simulink model "DLS_Controller_SW"  (Simulink 7.9)
settings: Solver=FixedStepDiscrete  StartTime=0.0  StopTime=10  RelTol=1e-3
PreLoadFcn:
  | DLS_Controller_SW_selfinit
settings Model: Creator=fguerin  LastModifiedBy=klindqvi  RecordCoverage=on
settings DataIOCC: ExternalInput=[t,u]  LimitDataPoints=off  SaveOutput=off  DSMLogging=off  SaveTime=off  SignalLoggingName=logsOut
settings OptimizationCC: InlineParams=on  InlineInvariantSignals=on  EnhancedBackFolding=on  ZeroExternalMemoryAtStartup=off  ZeroInternalMemoryAtStartup=off  EfficientFloat2IntCast=on  OptimizeModelRefInitCode=on  LifeSpan=1
settings DebuggingCC: SignalInfNanChecking=error  SignalRangeChecking=error  ReadBeforeWriteMsg=EnableAllAsError  WriteAfterWriteMsg=EnableAllAsError  WriteAfterReadMsg=EnableAllAsError  AlgebraicLoopMsg=error  ArtificialAlgebraicLoopMsg=error  SaveWithDisabledLinksMsg=error  SaveWithParameterizedLinksMsg=error  CheckExecutionContextPreStartOutputMsg=on  CheckExecutionContextRuntimeOutputMsg=on  BlockPriorityViolationMsg=error  SolverPrmCheckMsg=error  MultiTaskCondExecSysMsg=warning  MultiTaskRateTransMsg=warning  CheckMatrixSingularityMsg=error  IntegerOverflowMsg=error  ParameterUnderflowMsg=error  ParameterPrecisionLossMsg=error  ParameterTunabilityLossMsg=error  UnderSpecifiedDataTypeMsg=warning  UnnecessaryDatatypeConvMsg=warning  VectorMatrixConversionMsg=error  SFcnCompatibilityMsg=error  BusObjectLabelMismatch=error  RootOutportRequireBusObject=error  AssertControl=DisableAll  ModelReferenceIOMsg=error  ModelReferenceIOMismatchMessage=error  ModelReferenceCSMismatchMessage=warning  UnknownTsInhSupMsg=error  ModelReferenceDataLoggingMessage=error  ModelReferenceSymbolNameMessage=none  StrictBusMsg=ErrorOnBusTreatedAsVector
settings HardwareCC: ProdLargestAtomicInteger=Long  ProdLargestAtomicFloat=Double  ProdIntDivRoundTo=Zero  ProdEndianess=BigEndian  ProdHWDeviceType=Freescale->MPC5500
settings ModelReferenceCC: ModelReferenceNumInstancesAllowed=Single
settings SFSimCC: SimParseCustomCode=off
settings RTWCC: SystemTargetFile=ert.tlc  TemplateMakefile=ert_default_tmf  Description=Embedded Coder  GenerateReport=on  RTWVerbose=off  ProcessScript=ert_make_rtw_hook  IncludeHyperlinkInReport=on  LaunchReport=on  GenerateTraceInfo=on  GenerateTraceReport=on  GenerateTraceReportSl=on  GenerateTraceReportSf=on  GenerateTraceReportEml=on  GenerateCodeMetricsReport=on
settings MATStruct: className=rtw.pil.Bullseye  argsAllComponents=[]  excludedModels=[]  includeReferencedModels=off  includeTopModel=on  enabled=off
settings CodeAppCC: ForceParamTrailComments=on  IgnoreCustomStorageClasses=off  IgnoreTestpoints=on  MangleLength=4  InlinedPrmAccess=Macros  ReqsInCode=on
settings ERTTargetCC: CodeReplacementLibrary=ANSI_C  MultiwordLength=2048  GenerateSampleERTMain=on  SupportAbsoluteTime=off  SupportNonFinite=off  SupportComplex=off  PortableWordSizes=on  InlinedParameterPlacement=NonHierarchical  ERTCustomFileTemplate=example_file_process.tlc  ConvertIfToSwitch=off  SuppressUnreachableDefaultCases=off
settings ConfigComp: Description=Design Verifier Custom Configuration Component  DVMaxProcessTime=600  DVDisplayUnsatisfiableObjectives=on  DVAutomaticStubbing=off  DVOutputDir=C:\Work\Data\Pilots\P_PSA_ECoder_BenchMark_LaGarenne\source9b\deliverable\trunk\demos\VnV_example\Projects\ADL_Project/Simulink_Test_Generation/ADL_Sim  DVModelCoverageObjectives=MCDC  DVTestSuiteOptimization=CombinedObjectives  DVDataFileName=./Tests/$ModelName$_sldvdata  DVSaveHarnessModel=on  DVHarnessModelFileName=./Tests/$ModelName$_testHarness  DVModelReferenceHarness=on  DVSaveReport=on  DVReportFileName=ADL_Sim_SLDV.html

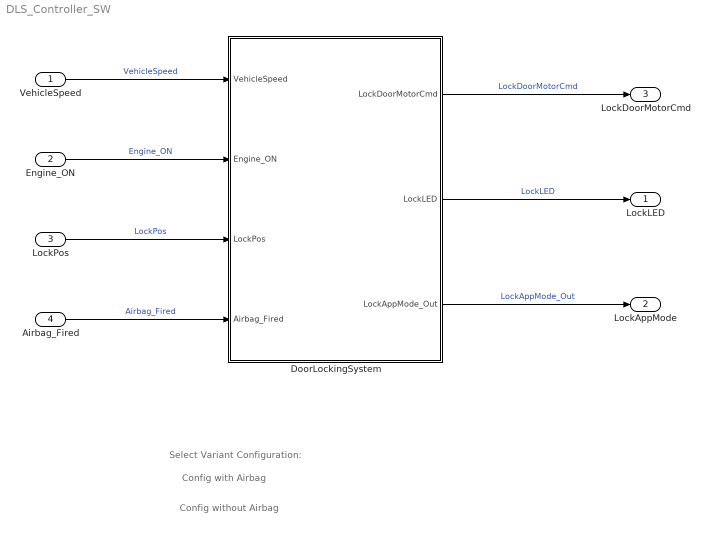
== system DLS_Controller_SW ==
  note: Select Variant Configuration:
  note: Config with Airbag
  note: Config without Airbag
  VehicleSpeed : Inport  PortDimensions=1  SampleTime=0.25
  Engine_ON : Inport  Port=2  PortDimensions=1  SampleTime=0.25
  LockPos : Inport  Port=3  SampleTime=0.25
  Airbag_Fired : Inport  Port=4  OutDataTypeStr=boolean  PortDimensions=1  SampleTime=0.25
  DoorLockingSystem : Subsystem
  LockLED : Outport  OutDataTypeStr=boolean  PortDimensions=1
  LockAppMode : Outport  Port=2
  LockDoorMotorCmd : Outport  Port=3
  wires:
  VehicleSpeed/1 -> DoorLockingSystem/1(VehicleSpeed)  "VehicleSpeed"
  Engine_ON/1 -> DoorLockingSystem/2(Engine_ON)  "Engine_ON"
  DoorLockingSystem/2(LockLED) -> LockLED/1  "LockLED"
  DoorLockingSystem/1(LockDoorMotorCmd) -> LockDoorMotorCmd/1  "LockDoorMotorCmd"
  LockPos/1 -> DoorLockingSystem/3(LockPos)  "LockPos"
  Airbag_Fired/1 -> DoorLockingSystem/4(Airbag_Fired)  "Airbag_Fired"
  DoorLockingSystem/3(LockAppMode_Out) -> LockAppMode/1  "LockAppMode_Out"

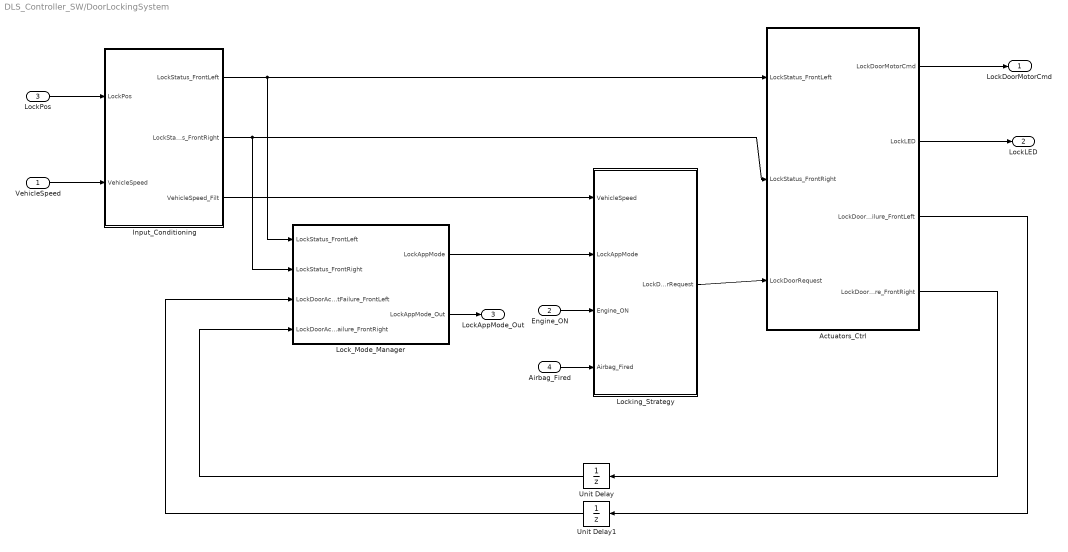
== system DLS_Controller_SW/DoorLockingSystem ==
  VehicleSpeed : Inport
  Engine_ON : Inport  Port=2  PortDimensions=1
  LockPos : Inport  Port=3
  Airbag_Fired : Inport  Port=4  OutDataTypeStr=boolean  PortDimensions=1
  Actuators_Ctrl : Subsystem
  Input_Conditioning : Subsystem
  Lock_Mode_Manager : Subsystem
  Locking_Strategy : Subsystem
  Unit Delay : UnitDelay  SampleTime=-1
  Unit Delay1 : UnitDelay  SampleTime=-1
  LockDoorMotorCmd : Outport
  LockLED : Outport  Port=2
  LockAppMode_Out : Outport  Port=3
  wires:
  VehicleSpeed/1 -> Input_Conditioning/2(VehicleSpeed)
  Engine_ON/1 -> Locking_Strategy/3(Engine_ON)
  Actuators_Ctrl/2(LockLED) -> LockLED/1
  LockPos/1 -> Input_Conditioning/1(LockPos)
  Locking_Strategy/1(LockDoorRequest) -> Actuators_Ctrl/3(LockDoorRequest)
  Actuators_Ctrl/1(LockDoorMotorCmd) -> LockDoorMotorCmd/1
  Lock_Mode_Manager/1(LockAppMode) -> Locking_Strategy/2(LockAppMode)
  Airbag_Fired/1 -> Locking_Strategy/4(Airbag_Fired)
  Input_Conditioning/3(VehicleSpeed_Filt) -> Locking_Strategy/1(VehicleSpeed)
  Input_Conditioning/1(LockStatus_FrontLeft) -> Actuators_Ctrl/1(LockStatus_FrontLeft), Lock_Mode_Manager/1(LockStatus_FrontLeft)
  Input_Conditioning/2(LockStatus_FrontRight) -> Actuators_Ctrl/2(LockStatus_FrontRight), Lock_Mode_Manager/2(LockStatus_FrontRight)
  Lock_Mode_Manager/2(LockAppMode_Out) -> LockAppMode_Out/1
  Actuators_Ctrl/3(LockDoorActFailure_FrontLeft) -> Unit Delay1/1
  Actuators_Ctrl/4(LockDoorActFailure_FrontRight) -> Unit Delay/1
  Unit Delay/1 -> Lock_Mode_Manager/4(LockDoorActFailure_FrontRight)
  Unit Delay1/1 -> Lock_Mode_Manager/3(LockDoorActFailure_FrontLeft)

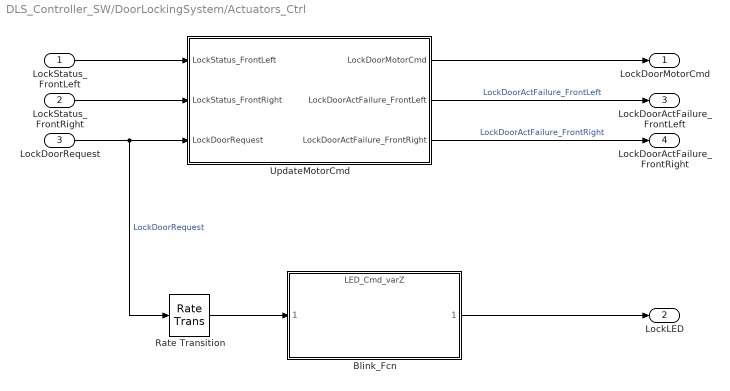
== system DLS_Controller_SW/DoorLockingSystem/Actuators_Ctrl ==
  LockStatus_FrontLeft : Inport
  LockStatus_FrontRight : Inport  Port=2
  LockDoorRequest : Inport  Port=3
  Blink_Fcn : ModelReference  ModelNameDialog=LED_Cmd_varZ  SimulationMode=Normal  ModelReferenceVersion=1.341  CopyOfModelName=LED_Cmd_varZ  DefaultDataLogging=off
  Rate Transition : RateTransition  Integrity=off  OutPortSampleTime=1
  UpdateMotorCmd : Subsystem
      settings: RTWFcnNameOpts=Use subsystem name  RTWFileNameOpts=User specified
  LockDoorMotorCmd : Outport
  LockLED : Outport  Port=2
  LockDoorActFailure_FrontLeft : Outport  Port=3
  LockDoorActFailure_FrontRight : Outport  Port=4
  wires:
  LockDoorRequest/1 -> UpdateMotorCmd/3(LockDoorRequest), Rate Transition/1  "LockDoorRequest"
  UpdateMotorCmd/1(LockDoorMotorCmd) -> LockDoorMotorCmd/1
  UpdateMotorCmd/2(LockDoorActFailure_FrontLeft) -> LockDoorActFailure_FrontLeft/1  "LockDoorActFailure_FrontLeft"
  LockStatus_FrontLeft/1 -> UpdateMotorCmd/1(LockStatus_FrontLeft)
  LockStatus_FrontRight/1 -> UpdateMotorCmd/2(LockStatus_FrontRight)
  UpdateMotorCmd/3(LockDoorActFailure_FrontRight) -> LockDoorActFailure_FrontRight/1  "LockDoorActFailure_FrontRight"
  Blink_Fcn/1 -> LockLED/1
  Rate Transition/1 -> Blink_Fcn/1

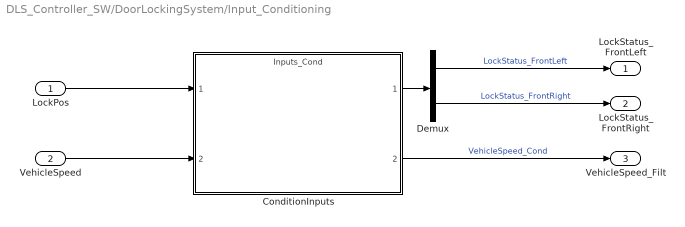
== system DLS_Controller_SW/DoorLockingSystem/Input_Conditioning ==
  LockPos : Inport
  VehicleSpeed : Inport  Port=2
  ConditionInputs : ModelReference  ModelNameDialog=Inputs_Cond  SimulationMode=Normal  ModelReferenceVersion=1.360  CopyOfModelName=Inputs_Cond  DefaultDataLogging=off
  Demux : Demux  Outputs=2
  LockStatus_FrontLeft : Outport
  LockStatus_FrontRight : Outport  Port=2
  VehicleSpeed_Filt : Outport  Port=3
  wires:
  LockPos/1 -> ConditionInputs/1
  VehicleSpeed/1 -> ConditionInputs/2
  ConditionInputs/2 -> VehicleSpeed_Filt/1  "VehicleSpeed_Cond"
  Demux/2 -> LockStatus_FrontRight/1  "LockStatus_FrontRight"
  ConditionInputs/1 -> Demux/1
  Demux/1 -> LockStatus_FrontLeft/1  "LockStatus_FrontLeft"

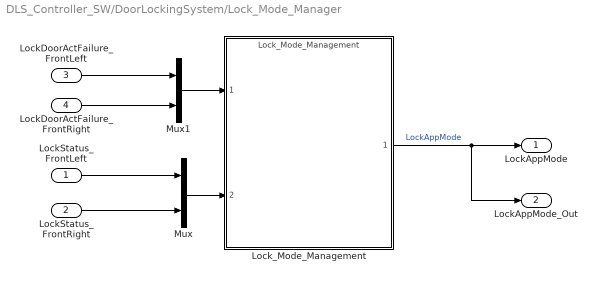
== system DLS_Controller_SW/DoorLockingSystem/Lock_Mode_Manager ==
  LockStatus_FrontLeft : Inport
  LockStatus_FrontRight : Inport  Port=2
  LockDoorActFailure_FrontLeft : Inport  Port=3
  LockDoorActFailure_FrontRight : Inport  Port=4
  Lock_Mode_Management : ModelReference  ModelNameDialog=Lock_Mode_Management  SimulationMode=Normal  ModelReferenceVersion=1.378  CopyOfModelName=Lock_Mode_Management  DefaultDataLogging=off
  Mux : Mux  Inputs=2
  Mux1 : Mux  Inputs=2
  LockAppMode : Outport
  LockAppMode_Out : Outport  Port=2
  wires:
  Lock_Mode_Management/1 -> LockAppMode/1, LockAppMode_Out/1  "LockAppMode"
  LockStatus_FrontLeft/1 -> Mux/1
  LockStatus_FrontRight/1 -> Mux/2
  Mux/1 -> Lock_Mode_Management/2
  LockDoorActFailure_FrontRight/1 -> Mux1/2
  Mux1/1 -> Lock_Mode_Management/1
  LockDoorActFailure_FrontLeft/1 -> Mux1/1

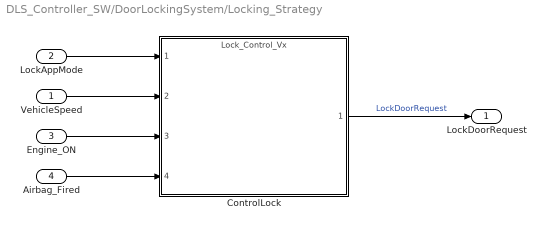
== system DLS_Controller_SW/DoorLockingSystem/Locking_Strategy ==
  VehicleSpeed : Inport
  LockAppMode : Inport  Port=2  PortDimensions=1
  Engine_ON : Inport  Port=3
  Airbag_Fired : Inport  Port=4  OutDataTypeStr=boolean  PortDimensions=1
  ControlLock : ModelReference  ModelNameDialog=Lock_Control_Vx  SimulationMode=Normal  Variant=on  ModelReferenceVersion=1.333  CopyOfModelName=Lock_Control_Vx  DefaultDataLogging=off
      settings: AttributesFormatString=%<ActiveVariant>
  LockDoorRequest : Outport
  wires:
  ControlLock/1 -> LockDoorRequest/1  "LockDoorRequest"
  VehicleSpeed/1 -> ControlLock/2
  Engine_ON/1 -> ControlLock/3
  Airbag_Fired/1 -> ControlLock/4
  LockAppMode/1 -> ControlLock/1

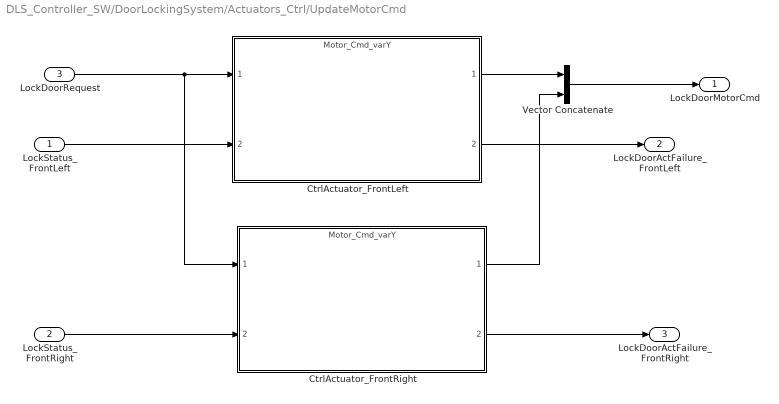
== system DLS_Controller_SW/DoorLockingSystem/Actuators_Ctrl/UpdateMotorCmd ==
  LockStatus_FrontLeft : Inport
  LockStatus_FrontRight : Inport  Port=2
  LockDoorRequest : Inport  Port=3
  CtrlActuator_FrontLeft : ModelReference  ModelNameDialog=Motor_Cmd_varY  SimulationMode=Normal  ModelReferenceVersion=1.46  CopyOfModelName=Motor_Cmd_varY  DefaultDataLogging=off
  CtrlActuator_FrontRight : ModelReference  ModelNameDialog=Motor_Cmd_varY  ModelReferenceVersion=1.46  CopyOfModelName=Motor_Cmd_varY  DefaultDataLogging=off
  Vector Concatenate : Concatenate
  LockDoorMotorCmd : Outport
  LockDoorActFailure_FrontLeft : Outport  Port=2
  LockDoorActFailure_FrontRight : Outport  Port=3
  wires:
  LockDoorRequest/1 -> CtrlActuator_FrontLeft/1, CtrlActuator_FrontRight/1
  CtrlActuator_FrontLeft/1 -> Vector Concatenate/1
  CtrlActuator_FrontLeft/2 -> LockDoorActFailure_FrontLeft/1
  LockStatus_FrontRight/1 -> CtrlActuator_FrontRight/2
  CtrlActuator_FrontRight/2 -> LockDoorActFailure_FrontRight/1
  CtrlActuator_FrontRight/1 -> Vector Concatenate/2
  Vector Concatenate/1 -> LockDoorMotorCmd/1
  LockStatus_FrontLeft/1 -> CtrlActuator_FrontLeft/2
